simulink model "mpc_simulink_with_r_and_d"  (R2015a)
settings: Solver=ode45  SolverMode=SingleTasking  StartTime=0.0  StopTime=20  RelTol=1e-3
values from neighbouring files (symbols this model uses):
  plant = tf([2 3],[a 5 1])    [mpc_period_abitary_input.m]    (also in mpc_period_exp.m = tf([3],[a 1]); mpc_period_with_abitary_reference.m)
undefined symbols (not defined in the file or in its folder): simu
libraries: mpclib x1
settings Model: CovSFcnEnable=off  ExtModeTrigMode=oneshot  ExtModeArmWhenConnect=off  Creator=The MathWorks Inc.  LastModifiedBy=Xiaotian
settings DataIOCC: LimitDataPoints=off  SaveOutput=off  SignalLogging=off  DSMLogging=off  SaveTime=off  SignalLoggingName=sigsOut
settings OptimizationCC: BooleanDataType=off  ExpressionDepthLimit=2147483647  InitFltsAndDblsToZero=on
settings DebuggingCC: SaveWithParameterizedLinksMsg=none  UnderspecifiedInitializationDetection=Classic  MergeDetectMultiDrivingBlocksExec=none  SignalResolutionControl=TryResolveAllWithWarning  MultiTaskDSMMsg=warning  MultiTaskCondExecSysMsg=none  IntegerOverflowMsg=none  FcnCallInpInsideContextMsg=UseLocalSettings  StateNameClashWarn=warning  IntegerSaturationMsg=none
settings HardwareCC: TargetUnknown=on
settings GRTTargetCC: TargetFcnLib=ansi_tfl_tmw.mat  CombineOutputUpdateFcns=off  GRTInterface=on

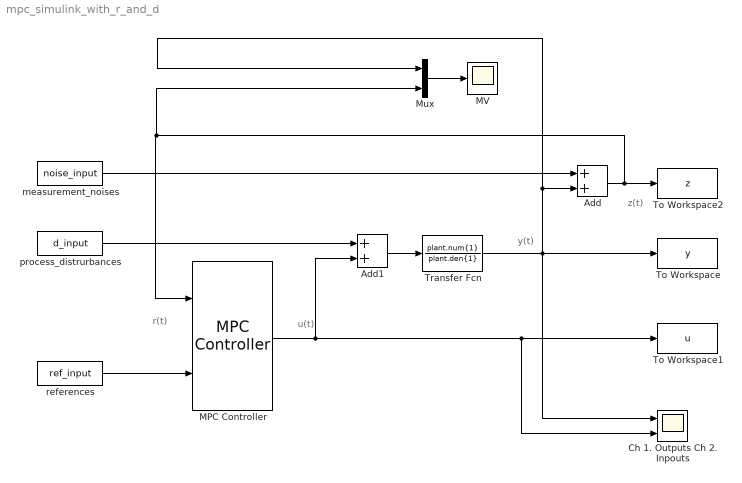
== system mpc_simulink_with_r_and_d ==
  note: r(t)
  note: u(t)
  note: y(t)
  note: z(t)
  Add : Sum
  Add1 : Sum
  Ch 1. Outputs Ch 2. Inpouts : Scope  NumInputPorts=2
      settings: TimeRange=10  YMin=-29.95~-11  YMax=-29.6~-9  DataFormat=Structure  SampleInput=on  SampleTime=simu.samlping_time
  MPC Controller : mpclib/MPC Controller  mpcobj=mpcobj  x0=[]  is_multiple=0  enable_value=0  n_mv=1  n_mo=1  n_md=0  n_ts=0.1  is_designfromscratch=0  return_u0=off  ref_from_ws=off  ref_signal_name=[]  ref_preview=on  md_from_ws=off  md_signal_name=[]  md_preview=on  from_project=off  project_file=MPCtask.mat  md_inport=off  mv_inport=off  cost_outport=off  return_sequence=off  return_qpstatus=off  return_state=off  state_inport=off  lims_inport=off  ywt_inport=off  uwt_inport=off  duwt_inport=off  rhoeps_inport=off  uref_inport=off  BlockDataType=double  SampleTimeInherited=off  switch_inport=off
  MV : Scope
      settings: TimeRange=10  YMin=-1.5  YMax=1.75  DataFormat=Structure
  Mux : Mux  Inputs=2
  To Workspace : ToWorkspace  VariableName=y  SampleTime=simu.samlping_time
      settings: MaxDataPoints=Inf
  To Workspace1 : ToWorkspace  VariableName=u  SampleTime=simu.samlping_time
      settings: MaxDataPoints=Inf
  To Workspace2 : ToWorkspace  VariableName=z  SampleTime=simu.samlping_time
      settings: MaxDataPoints=Inf
  Transfer Fcn : TransferFcn  Numerator=plant.num{1}  Denominator=plant.den{1}
  measurement_noises : FromWorkspace  VariableName=noise_input  SampleTime=0
  process_distrurbances : FromWorkspace  VariableName=d_input  SampleTime=0
  references : FromWorkspace  VariableName=ref_input  SampleTime=0
  wires:
  MPC Controller/1 -> Add1/2, To Workspace1/1, Ch 1. Outputs Ch 2. Inpouts/2
  Transfer Fcn/1 -> Ch 1. Outputs Ch 2. Inpouts/1, Mux/1, Add/2, To Workspace/1
  references/1 -> MPC Controller/2
  Add/1 -> To Workspace2/1, Mux/2, MPC Controller/1
  measurement_noises/1 -> Add/1
  Add1/1 -> Transfer Fcn/1
  process_distrurbances/1 -> Add1/1
  Mux/1 -> MV/1
